simulink model "sldemo_auto_climate_elec"  (R2021b)
settings: Solver=ode23t  StartTime=0.0  StopTime=1  MaxStep=1e-4  RelTol=1e-4  AbsTol=1e-4  EnableMultiTasking=on
undefined symbols (not defined in the file or in its folder): ee
libraries: fl_lib x15, nesl_utility x10, ee_lib x9, commchan3 x3, slpidlib x1, simulink x1
(part 1 of 2)
settings Model: Creator=The MathWorks, Inc.  LastModifiedBy=dev
settings SolverCC: AutoScaleAbsTol=off  AlgebraicLoopSolver=TrustRegion
settings DataIOCC: SaveFormat=Array  ReturnWorkspaceOutputs=off  SignalLoggingName=sigsOut
settings OptimizationCC: ExpressionDepthLimit=2147483647  InitFltsAndDblsToZero=on  EfficientMapNaN2IntZero=off  LifeSpan=inf
settings DebuggingCC: AlgebraicLoopMsg=error  SaveWithParameterizedLinksMsg=none  UnderspecifiedInitializationDetection=Classic  MergeDetectMultiDrivingBlocksExec=none  SignalResolutionControl=TryResolveAllWithWarning  MultiTaskDSMMsg=warning  MultiTaskCondExecSysMsg=none  FcnCallInpInsideContextMsg=warning  StateNameClashWarn=warning  SFUnexpectedBacktrackingDiag=warning  SFNoUnconditionalDefaultTransitionDiag=warning  SFExecutionAtInitializationDiag=none  SFMachineParentedDataDiag=warning  ArithmeticOperatorsInVariantConditions=warning
settings HardwareCC: ProdBitPerPointer=32  ProdBitPerSizeT=32  ProdBitPerPtrDiffT=32  ProdLargestAtomicFloat=None  ProdIntDivRoundTo=Undefined  ProdEndianess=Unspecified  ProdWordSize=32  ProdHWDeviceType=32-bit Generic
settings ModelReferenceCC: PropagateSignalLabelsOutOfModel=off
settings SFSimCC: SimUseLocalCustomCode=off  CustomCodeUndefinedFunction=UseInterfaceOnly
settings RTWCC: RTWUseLocalCustomCode=off
settings CodeAppCC: StateflowObjectComments=on
settings GRTTargetCC: TargetFcnLib=ansi_tfl_tmw.mat  TargetLangStandard=C89/C90 (ANSI)  CombineOutputUpdateFcns=off  GRTInterface=on
settings ConfigComp: CovMetricSettings=dw  CovSaveCumulativeToWorkspaceVar=on  CovSaveSingleToWorkspaceVar=on  CovExternalEMLEnable=off
settings SimscapeCC: SimscapeLogType=all  SimscapeLogName=simlog_sldemo_auto_climate_elec  SimscapeLogLimitData=off

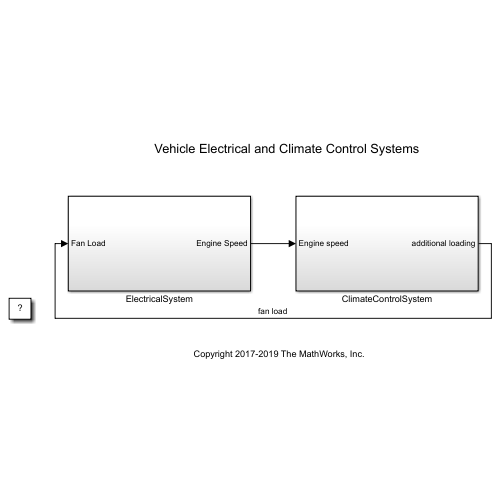
[thumbnail: Simulink's stored preview of the top-level diagram]
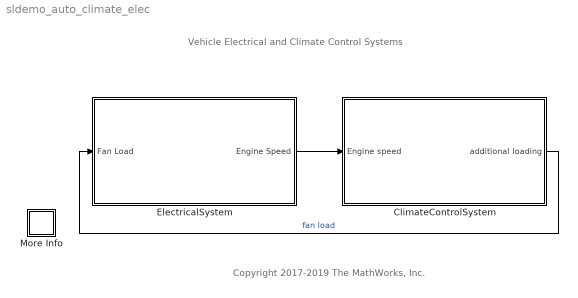
== system sldemo_auto_climate_elec ==
  note: Vehicle Electrical and Climate Control Systems
  note: Copyright 2017-2019 The MathWorks, Inc.
  ClimateControlSystem : Subsystem
  ElectricalSystem : Subsystem
  More Info : Subsystem
      settings: OpenFcn=showExample('simulink_automotive/VehicleElectricalAndClimateControlSystemsExample')
      mask Display: disp('?')
  wires:
  ElectricalSystem/1(Engine Speed) -> ClimateControlSystem/1(Engine speed)
  ClimateControlSystem/1(additional loading) -> ElectricalSystem/1(Fan Load)  "fan load"

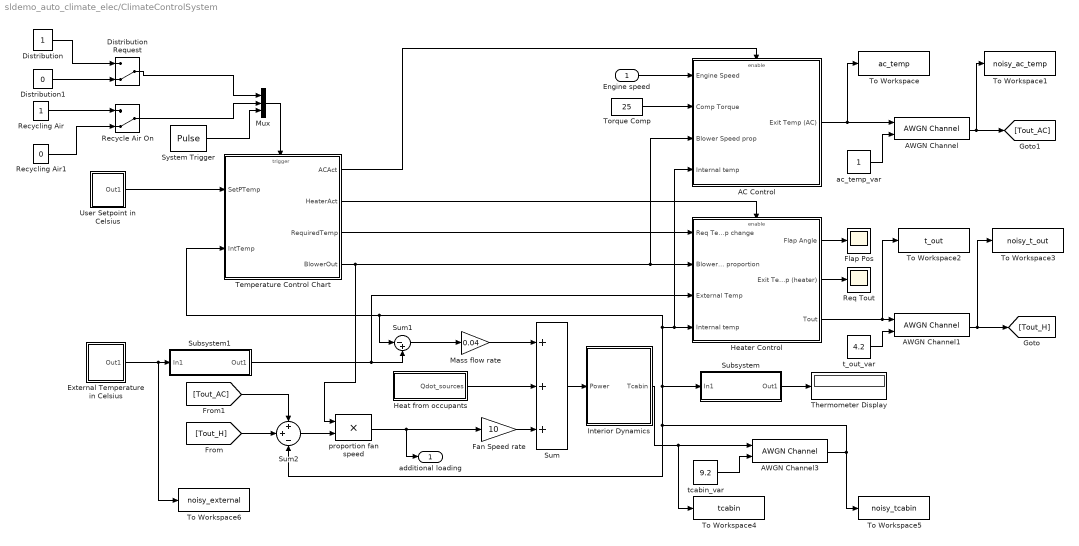
== system sldemo_auto_climate_elec/ClimateControlSystem ==
  Engine speed : Inport
  AC Control : Subsystem  TreatAsAtomicUnit=on
  AWGN Channel : commchan3/AWGN Channel  InputProcessing=Columns as channels (frame based)  seed=67  noiseMode=Variance from port  EbNodB=10  EsNodB=10  SNRdB=10  bitsPerSym=1  Ps=1  Tsym=1  variance=1
  AWGN Channel1 : commchan3/AWGN Channel  InputProcessing=Columns as channels (frame based)  seed=67  noiseMode=Variance from port  EbNodB=10  EsNodB=10  SNRdB=10  bitsPerSym=1  Ps=1  Tsym=1  variance=1
  AWGN Channel3 : commchan3/AWGN Channel  InputProcessing=Columns as channels (frame based)  seed=67  noiseMode=Variance from port  EbNodB=10  EsNodB=10  SNRdB=10  bitsPerSym=1  Ps=1  Tsym=1  variance=1
  "Distribution " : Constant
  Distribution Request : ManualSwitch  CurrentSetting=0
  "Distribution1 " : Constant  Value=0
  External Temperature in Celsius : Subsystem  mask(variable){x=18}
      mask prompts: x "Enter the external temperature"
      mask Display: disp(x);
  Fan Speed rate : Gain  Gain=10  SaturateOnIntegerOverflow=on  OutDataTypeStr=Inherit: Same as input  ParamDataTypeStr=Inherit: Same as input
  Flap Pos : Scope
  Heat from occupants : Subsystem  mask(Heat from occupants){N=1}
      mask prompts: N "Number of occupants:"
      settings: AttributesFormatString=No. of occupants: %<N>
      mask Display: disp('Heat Sources')
  Heater Control : Subsystem  TreatAsAtomicUnit=on
  Interior Dynamics : Subsystem  mask(Vehicle Cabin Dynamics){}
      mask Display: image('$imagefile') % use "Edit Image" on toolstrip to change
  Mass flow rate : Gain  Gain=0.04  SaturateOnIntegerOverflow=on  OutDataTypeStr=Inherit: Same as input  ParamDataTypeStr=Inherit: Same as input
  Mux : Mux  Inputs=3
  Recycle Air On : ManualSwitch  CurrentSetting=0
  Recycling Air : Constant
  Recycling Air1 : Constant  Value=0
  Req Tout : Scope
  Subsystem : Subsystem
      mask Display: disp('Kelvin to Celsius')
  Subsystem1 : Subsystem
      mask Display: disp('Celsius to Kelvin')
  Sum : Sum  Inputs=+++  InputSameDT=on  SaturateOnIntegerOverflow=on  OutDataTypeStr=Inherit: Same as first input
  Sum1 : Sum  Inputs=|-+  InputSameDT=on  SaturateOnIntegerOverflow=on  OutDataTypeStr=Inherit: Same as first input
  Sum2 : Sum  Inputs=++-  InputSameDT=on  SaturateOnIntegerOverflow=on  OutDataTypeStr=Inherit: Same as first input
  System Trigger : DiscretePulseGenerator  PulseType=Time based  Period=1/60  PulseWidth=50
  Temperature Control Chart : Stateflow chart  TreatAsAtomicUnit=on
  Thermometer Display : Display
  To Workspace : ToWorkspace  VariableName=ac_temp  SampleTime=-1
      settings: Save2DSignal=2-D array (concatenate along first dimension)
  To Workspace1 : ToWorkspace  VariableName=noisy_ac_temp  SampleTime=-1
      settings: Save2DSignal=2-D array (concatenate along first dimension)
  To Workspace2 : ToWorkspace  VariableName=t_out  SampleTime=-1
      settings: Save2DSignal=2-D array (concatenate along first dimension)
  To Workspace3 : ToWorkspace  VariableName=noisy_t_out  SampleTime=-1
      settings: Save2DSignal=2-D array (concatenate along first dimension)
  To Workspace4 : ToWorkspace  VariableName=tcabin  SampleTime=-1
      settings: Save2DSignal=2-D array (concatenate along first dimension)
  To Workspace5 : ToWorkspace  VariableName=noisy_tcabin  SampleTime=-1
      settings: Save2DSignal=2-D array (concatenate along first dimension)
  To Workspace6 : ToWorkspace  VariableName=noisy_external  SampleTime=-1
      settings: Save2DSignal=2-D array (concatenate along first dimension)
  Torque Comp : Constant  Value=25
  User Setpoint in Celsius : Subsystem  mask{USet=40}
      mask prompts: USet "Enter the Temperature you require"
      mask Display: disp(USet)
  ac_temp_var : Constant
  proportion fan speed : Product  InputSameDT=on  SaturateOnIntegerOverflow=on  OutDataTypeStr=Inherit: Same as first input
  t_out_var : Constant  Value=4.2
  tcabin_var : Constant  Value=9.2
  additional loading : Outport  VectorParamsAs1DForOutWhenUnconnected=off
  wires:
  Sum/1 -> Interior Dynamics/1(Power)
  Mux/1 -> Temperature Control Chart/Trigger
  Engine speed/1 -> AC Control/1(Engine Speed)
  AC Control/1(Exit Temp (AC)) -> To Workspace/1, AWGN Channel/1
  Temperature Control Chart/3(RequiredTemp) -> Heater Control/1(Req Temp change)
  Torque Comp/1 -> AC Control/2(Comp Torque)
  [Tout_AC] -> Sum2/1
  Temperature Control Chart/1(" ACAct") -> AC Control/Enable
  [Tout_H] -> Sum2/2
  Heater Control/3(Tout) -> To Workspace2/1, AWGN Channel1/1
  Heater Control/2(Exit Temp (heater)) -> Req Tout/1
  Heater Control/1(Flap Angle) -> Flap Pos/1
  Temperature Control Chart/2(" HeaterAct") -> Heater Control/Enable
  proportion fan speed/1 -> Fan Speed rate/1, additional loading/1
  Temperature Control Chart/4(BlowerOut) -> proportion fan speed/1, Heater Control/2(Blower Speed proportion), AC Control/3(Blower Speed prop)
  Sum2/1 -> proportion fan speed/2
  Fan Speed rate/1 -> Sum/3
  Subsystem1/1(Out1) -> Sum1/2, Heater Control/3(External Temp)
  Sum1/1 -> Mass flow rate/1
  Mass flow rate/1 -> Sum/1
  Heat from occupants/1(Qdot_sources) -> Sum/2
  Subsystem/1(Out1) -> Thermometer Display/1
  AWGN Channel3/1 -> To Workspace5/1, Subsystem/1(In1), Sum1/1, Temperature Control Chart/2(IntTemp), Heater Control/4(Internal temp), AC Control/4(Internal temp), Sum2/3
  System Trigger/1 -> Mux/3
  Recycle Air On/1 -> Mux/2
  Recycling Air/1 -> Recycle Air On/1
  User Setpoint in Celsius/1(Out1) -> Temperature Control Chart/1(SetPTemp)
  Recycling Air1/1 -> Recycle Air On/2
  "Distribution1 "/1 -> Distribution Request/2
  "Distribution "/1 -> Distribution Request/1
  Distribution Request/1 -> Mux/1
  AWGN Channel/1 -> To Workspace1/1, [Tout_AC]
  ac_temp_var/1 -> AWGN Channel/2
  AWGN Channel1/1 -> To Workspace3/1, [Tout_H]
  t_out_var/1 -> AWGN Channel1/2
  External Temperature in Celsius/1(Out1) -> To Workspace6/1, Subsystem1/1(In1)
  tcabin_var/1 -> AWGN Channel3/2
  Interior Dynamics/1("Tcabin ") -> AWGN Channel3/1, To Workspace4/1

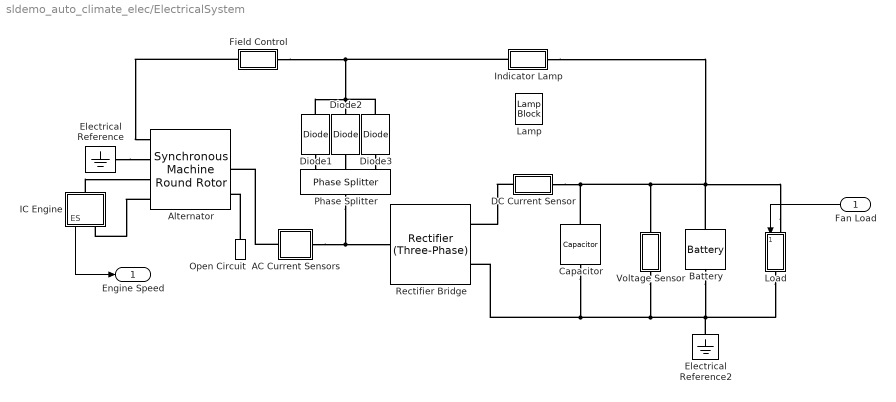
== system sldemo_auto_climate_elec/ElectricalSystem ==
  Fan Load : Inport
  AC Current Sensors : Subsystem
  Alternator : ee_lib/Electromechanical/Synchronous/Synchronous Machine Round Rotor  port_option=ee.enum.threePhasePort.composite  SRated=750 V*A  VRated=20 V  FRated=60 Hz  nPolePairs=3  param_option=ee.enum.sm.parameterization.fundamental  fieldCircuitParameterization_option=1  baseEfd=4.5 V  baseIfd=1300 A  zero_sequence=ee.enum.park.zerosequence.include  axes_param=ee.enum.rotorangle.daxis  Ladu=12.8  Laqu=12.48  L0=0.6  Ll=0.6  Ra=0.64  Lfd=1.32  Rfd=0.48  L1d=0.96  R1d=1.12  L1q=1.04  R1q=0.192  L2q=1.12  R2q=0.048  Xl=0.15  Xd=1.81  Xq=1.76  X0=0.15  Xdd=0.3  Xqd=0.65  Xddd=0.23  Xqdd=0.25  d_option=ee.enum.circuit.open  Td0d=8 s  Tdd=1.3260 s  Td0dd=0.03 s  Tddd=0.0230 s  q_option=ee.enum.circuit.open  Tq0d=1 s  Tqd=0.3693 s  Tq0dd=0.07 s  Tqdd=0.0269 s  saturation_option=0  saturation_ifd=[0, .48, .76, 1.38, 1.79]  saturation_Vag=[0, .8, 1.08, 1.31, 1.4]  initialization_option=1  source_type=ee.enum.sm.load_flow_source_type.Swing  Vmag0=1 V  Vang0=0 deg  Pt0=0 V*A  Qt0=0 V*A  minimum_pu=0.95  phase_search_range=[-30, 30] deg  gmin=1e-6 S  connection_option=int32(ee.enum.Connection.wye)  num_q_dampers=2  rotor_offset=-pi / 2 rad  pu_psid_specify=on  pu_psid_priority=High  pu_psid=0  pu_psid_nominal_specify=off  pu_psid_nominal_unit=1  pu_psid_nominal_value=1  pu_psiq_specify=on  pu_psiq_priority=High  pu_psiq=0  pu_psiq_nominal_specify=off  pu_psiq_nominal_unit=1  pu_psiq_nominal_value=1  pu_psifd_specify=on  pu_psifd_priority=High  pu_psifd=0  pu_psifd_nominal_specify=off  pu_psifd_nominal_unit=1  pu_psifd_nominal_value=1  pu_psi1d_specify=on  pu_psi1d_priority=High  pu_psi1d=0  pu_psi1d_nominal_specify=off  pu_psi1d_nominal_unit=1  pu_psi1d_nominal_value=1  pu_psi1q_specify=on  pu_psi1q_priority=High  pu_psi1q=0  pu_psi1q_nominal_specify=off  pu_psi1q_nominal_unit=1  pu_psi1q_nominal_value=1  pu_psi2q_specify=on  pu_psi2q_priority=High  pu_psi2q=0  pu_psi2q_nominal_specify=off  pu_psi2q_nominal_unit=1  pu_psi2q_nominal_value=1  angular_position_diff_specify=on  angular_position_diff_priority=High  angular_position_diff=0 deg  angular_position_diff_nominal_specify=off  angular_position_diff_nominal_unit=deg  angular_position_diff_nominal_value=1  Tmeas=298.15 K  alpha=3.93e-3 1/K  stator_thermal_mass=100 J/K  rotor_thermal_mass=200 J/K  temperatureA_specify=off  temperatureA_priority=High  temperatureA=25 degC  temperatureA_nominal_specify=off  temperatureA_nominal_unit=degC  temperatureA_nominal_value=1  temperatureB_specify=off  temperatureB_priority=High  temperatureB=25 degC  temperatureB_nominal_specify=off  temperatureB_nominal_unit=degC  temperatureB_nominal_value=1  temperatureC_specify=off  temperatureC_priority=High  temperatureC=25 degC  temperatureC_nominal_specify=off  temperatureC_nominal_unit=degC  temperatureC_nominal_value=1  temperatureR_specify=off  temperatureR_priority=High  temperatureR=25 degC  temperatureR_nominal_specify=off  temperatureR_nominal_unit=degC  temperatureR_nominal_value=1
      settings: SourceProductBaseCode=PS  InternalSimscapePortConfiguration="{\"Bottom\":[],\"Left\":[{\"id\":\"fd_p\",\"label\":\"fd+\",\"type\":\"foundation.electrical.electrical\"},{\"id\":\"fd_n\",\"label\":\"fd-\",\"type\":\"foundation.electrical.electrical\"},{\"id\":\"R\",\"label\":\"R\",\"type\":\"foundation.mechanical.rotational.rotational\"},{\"id\":\"C\",\"label\":\"C\",\"type\":\"foundation.mechanical.rotational.rotational\"}],\"Right\":[{\"id\":\"pu_output\",\"label\":\"pu\",\"type\":\"output\"},{\"id\":\"N\",\"label\":\"~\",\"type\":\"foundation.electrical.three_phase\"},{\"id\":\"n\",\"label\":\"n\",\"type\":\"foundation.electrical.electrical\"}],\"Top\":[]}"
  Battery : ee_lib/Sources/Battery  Vnom=12 V  prm_dir=1  R1_dis=2 Ohm  R1_ch=2 Ohm  R1=0.5 Ohm  prm_AH=2  AH=50 hr*A  V1=11.5 V  AH1=25 hr*A  prm_R2=1  R2=2000 Ohm  prm_dyn=1  Rp1=0.005 Ohm  tau1=30 s  Rp2=0.005 Ohm  tau2=30 s  Rp3=0.005 Ohm  tau3=30 s  Rp4=0.005 Ohm  tau4=30 s  Rp5=0.005 Ohm  tau5=30 s  prm_fade=1  N_fade=100  AH_fade=45 hr*A  R1_fade=2.02 Ohm  R1_ch_fade=2.02 Ohm  V1_fade=10.35 V  prm_age=1  prm_age_OCV=1  OCV_age=0.9  SOC_age=60  delta_time_age_vec=[0] d  temperature_age_vec=[273] K  OCV_scaling_age=2.2134e6  OCV_offset_age=1.632e6  temp_exp_age=0.515833569 V  t_exp_age=0.75  i_specify=off  i_priority=None  i=0 A  i_nominal_specify=off  i_nominal_unit=A  i_nominal_value=1  v_specify=off  v_priority=None  v=0 V  v_nominal_specify=off  v_nominal_unit=V  v_nominal_value=1  charge_specify=on  charge_priority=High  charge=50*0.80 hr*A  charge_nominal_specify=off  charge_nominal_unit=hr*A  charge_nominal_value=1  num_cycles_specify=off  num_cycles_priority=High  num_cycles=0  num_cycles_nominal_specify=off  num_cycles_nominal_unit=1  num_cycles_nominal_value=1  Tmeas=298.15 K  Tmeas_age=298.15 K  Vnom_T2=12 V  R1_T2=2.2 Ohm  R1_T2_dis=2.2 Ohm  R1_T2_ch=2.2 Ohm  V1_T2=11.4 V  R2_T2=2200 Ohm  Rp1_T2=0.005 Ohm  tau1_T2=30 s  Rp2_T2=0.005 Ohm  tau2_T2=30 s  Rp3_T2=0.005 Ohm  tau3_T2=30 s  Rp4_T2=0.005 Ohm  tau4_T2=30 s  Rp5_T2=0.005 Ohm  tau5_T2=30 s  Tmeas2=273.15 K  thermal_mass=30000 J/K  temperature_specify=off  temperature_priority=High  temperature=298.15 K  temperature_nominal_specify=off  temperature_nominal_unit=K  temperature_nominal_value=1
  Capacitor : fl_lib/Electrical/Electrical Elements/Capacitor  c=50e-6 F  r=0 Ohm  g=1e-6 1/Ohm  i_specify=off  i_priority=None  i=0 A  i_nominal_specify=off  i_nominal_unit=A  i_nominal_value=1  v_specify=off  v_priority=None  v=0 V  v_nominal_specify=off  v_nominal_unit=V  v_nominal_value=1  vc_specify=on  vc_priority=High  vc=12 V  vc_nominal_specify=off  vc_nominal_unit=V  vc_nominal_value=1
  DC Current Sensor : Subsystem
  Diode1 : ee_lib/Semiconductors & Converters/Diode  ModelType=ee.enum.diode.modelType.pwl  TableType=ee.enum.diode.tableType.IfMat  IfMat=[.07, .12, .19, 1.75, 4.24, 7.32, 11.2; .16, .3, .72, 2.14, 5.02, 8.35, 13.12] A  VfMat=[.9, 1.15, 1.25, 1.5, 1.75, 2.17, 2.6, 2.85; .58, .68, .75, 1.1, 1.38, 1.77, 2.27, 2.7] V  TjVec=[25, 125] degC  VfVec=[.5, .7, .9, 1.3, 1.7, 2.1, 2.5] V  IfVec=[.1, .2, .5, 1, 2, 4, 7, 10] A  Vf=0.8 V  Ron=0.001 Ohm  Goff=1e-5 1/Ohm  prmExp=ee.enum.diode.expParam.useTwo  I12=[.0137, .545] A  V12=[.6, .7] V  RS=0 Ohm  Tmeas=25 degC  IS=1e-12 A  ec=1  I1=0.0137 A  V1=0.6 V  N_series=1  N_parallel=1  Rz=0.3 Ohm  BV=inf V  C_param=ee.enum.diode.capParam.fixed  CJ=0 pF  CJ0=5 pF  Vvec=[.1, 10, 100] V  Cvec=[3.5, 1, .4] pF  VJ=1 V  Mgrad=0.5  FC=0.5  Q_param=ee.enum.diode.recoveryParam.off  iRM=-7.15 A  iF=4 A  didt=-750 A/us  trr_factor=3  trr=115 ns  Qrr=1500 s*uA  Vr=-600 V  Ls=150 nH  Erec=0.03 J  TT=50 ns  tau=100 ns  T_param=ee.enum.diode.temperatureParam.off  Tdevice=25 degC  I1_T2=0.245 A  V1_T2=0.5 V  IS_T2=1.25e-7 A  Tmeas2=125 degC  XTI_param=ee.enum.diode.xtiParam.pn  XTI=3  EG_param=ee.enum.diode.egapParam.material_si  EG=1.11 eV  dBVdT=0 V/K  enable_faults=simscape.enum.onoff.off  fault_action=simscape.enum.assert.action.none  fault_types=ee.enum.diode.faults.open  tau_fault=1e-3 s  IfMat_faulted=[.07, .12, .19, 1.75, 4.24, 7.32, 11.2; .16, .3, .72, 2.14, 4.02, 6.35, 9.12] A  VfMat_faulted=[.9, 1.15, 1.25, 1.5, 1.75, 2.17, 2.6, 2.85; .58, .68, .75, 1.1, 1.38, 1.77, 2.27, 2.7] V  VfVec_faulted=[.5, .7, .9, 1.3, 1.7, 2.1, 2.5] V  IfVec_faulted=[.1, .2, .5, 1, 2, 4, 7, 10] A  Ropen_faulted=1000 Ohm  Gshort_faulted=1000 1/Ohm  Vf_faulted=0.6 V  Ron_faulted=0.3 Ohm  Goff_faulted=1e-8 S  I12_faulted=[.0137, .545] A  V12_faulted=[.6, .7] V  IS_faulted=1e-12 A  ec_faulted=1  I1_faulted=0.0137 A  V1_faulted=0.6 V  RS_faulted=0 Ohm  Rz_faulted=0.3 Ohm  BV_faulted=inf V  Cscale_faulted=100  enable_temporal_fault=simscape.enum.onoff.off  t_fault=inf s  enable_behavioral_fault=simscape.enum.onoff.off  max_permissible_voltage=inf V  n_fail_on_voltage=1  max_permissible_current=inf A  t_fail_on_current=1 s  max_permissible_dVdt=inf V/s  i_specify=off  i_priority=None  i=0 A  i_nominal_specify=off  i_nominal_unit=A  i_nominal_value=1  v_specify=off  v_priority=None  v=0 V  v_nominal_specify=off  v_nominal_unit=V  v_nominal_value=1  i_diode_specify=off  i_diode_priority=None  i_diode=0 A  i_diode_nominal_specify=off  i_diode_nominal_unit=A  i_diode_nominal_value=1  v_diode_specify=off  v_diode_priority=None  v_diode=0 V  v_diode_nominal_specify=off  v_diode_nominal_unit=V  v_diode_nominal_value=1  i_capacitor_specify=off  i_capacitor_priority=None  i_capacitor=0 A  i_capacitor_nominal_specify=off  i_capacitor_nominal_unit=A  i_capacitor_nominal_value=1  v_capacitor_specify=off  v_capacitor_priority=None  v_capacitor=0 V  v_capacitor_nominal_specify=off  v_capacitor_nominal_unit=V  v_capacitor_nominal_value=1  power_dissipated_specify=off  power_dissipated_priority=None  power_dissipated=0 W  power_dissipated_nominal_specify=off  power_dissipated_nominal_unit=W  power_dissipated_nominal_value=1  max_permissible_temperature=inf K  t_fail_on_temperature=1 s  thermal_network_parameterization=ee.enum.thermalNetworkTopology.junctionCase  Rth=[0, 10] K/W  Rth_Cauer=[1, 3, 10] K/W  Rth_Foster=[4, 6] K/W  thermal_mass_parameterization=ee.enum.thermalNetwork.timeconstant  thermal_mass=[0, 1] J/K  thermal_mass_Cauer=[.1, .3, 1] J/K  thermal_mass_Foster=[1.5, 3] J/K  thermal_time_constant=[0, 10] s  thermal_time_constant_Cauer=[1, 3, 10] s  thermal_time_constant_Foster=[6, 18] s  thermal_mass_initial_temperatures=[25, 25] degC  thermal_mass_initial_temperatures_Cauer=[25, 25, 25] degC  steadyState_Foster=simscape.enum.onoff.on  Tvec_initial_Foster=[25, 25, 25, 25] degC
  Diode2 : ee_lib/Semiconductors & Converters/Diode  ModelType=ee.enum.diode.modelType.pwl  TableType=ee.enum.diode.tableType.IfMat  IfMat=[.07, .12, .19, 1.75, 4.24, 7.32, 11.2; .16, .3, .72, 2.14, 5.02, 8.35, 13.12] A  VfMat=[.9, 1.15, 1.25, 1.5, 1.75, 2.17, 2.6, 2.85; .58, .68, .75, 1.1, 1.38, 1.77, 2.27, 2.7] V  TjVec=[25, 125] degC  VfVec=[.5, .7, .9, 1.3, 1.7, 2.1, 2.5] V  IfVec=[.1, .2, .5, 1, 2, 4, 7, 10] A  Vf=0.8 V  Ron=0.001 Ohm  Goff=1e-5 1/Ohm  prmExp=ee.enum.diode.expParam.useTwo  I12=[.0137, .545] A  V12=[.6, .7] V  RS=0 Ohm  Tmeas=25 degC  IS=1e-12 A  ec=1  I1=0.0137 A  V1=0.6 V  N_series=1  N_parallel=1  Rz=0.3 Ohm  BV=inf V  C_param=ee.enum.diode.capParam.fixed  CJ=0 pF  CJ0=5 pF  Vvec=[.1, 10, 100] V  Cvec=[3.5, 1, .4] pF  VJ=1 V  Mgrad=0.5  FC=0.5  Q_param=ee.enum.diode.recoveryParam.off  iRM=-7.15 A  iF=4 A  didt=-750 A/us  trr_factor=3  trr=115 ns  Qrr=1500 s*uA  Vr=-600 V  Ls=150 nH  Erec=0.03 J  TT=50 ns  tau=100 ns  T_param=ee.enum.diode.temperatureParam.off  Tdevice=25 degC  I1_T2=0.245 A  V1_T2=0.5 V  IS_T2=1.25e-7 A  Tmeas2=125 degC  XTI_param=ee.enum.diode.xtiParam.pn  XTI=3  EG_param=ee.enum.diode.egapParam.material_si  EG=1.11 eV  dBVdT=0 V/K  enable_faults=simscape.enum.onoff.off  fault_action=simscape.enum.assert.action.none  fault_types=ee.enum.diode.faults.open  tau_fault=1e-3 s  IfMat_faulted=[.07, .12, .19, 1.75, 4.24, 7.32, 11.2; .16, .3, .72, 2.14, 4.02, 6.35, 9.12] A  VfMat_faulted=[.9, 1.15, 1.25, 1.5, 1.75, 2.17, 2.6, 2.85; .58, .68, .75, 1.1, 1.38, 1.77, 2.27, 2.7] V  VfVec_faulted=[.5, .7, .9, 1.3, 1.7, 2.1, 2.5] V  IfVec_faulted=[.1, .2, .5, 1, 2, 4, 7, 10] A  Ropen_faulted=1000 Ohm  Gshort_faulted=1000 1/Ohm  Vf_faulted=0.6 V  Ron_faulted=0.3 Ohm  Goff_faulted=1e-8 S  I12_faulted=[.0137, .545] A  V12_faulted=[.6, .7] V  IS_faulted=1e-12 A  ec_faulted=1  I1_faulted=0.0137 A  V1_faulted=0.6 V  RS_faulted=0 Ohm  Rz_faulted=0.3 Ohm  BV_faulted=inf V  Cscale_faulted=100  enable_temporal_fault=simscape.enum.onoff.off  t_fault=inf s  enable_behavioral_fault=simscape.enum.onoff.off  max_permissible_voltage=inf V  n_fail_on_voltage=1  max_permissible_current=inf A  t_fail_on_current=1 s  max_permissible_dVdt=inf V/s  i_specify=off  i_priority=None  i=0 A  i_nominal_specify=off  i_nominal_unit=A  i_nominal_value=1  v_specify=off  v_priority=None  v=0 V  v_nominal_specify=off  v_nominal_unit=V  v_nominal_value=1  i_diode_specify=off  i_diode_priority=None  i_diode=0 A  i_diode_nominal_specify=off  i_diode_nominal_unit=A  i_diode_nominal_value=1  v_diode_specify=off  v_diode_priority=None  v_diode=0 V  v_diode_nominal_specify=off  v_diode_nominal_unit=V  v_diode_nominal_value=1  i_capacitor_specify=off  i_capacitor_priority=None  i_capacitor=0 A  i_capacitor_nominal_specify=off  i_capacitor_nominal_unit=A  i_capacitor_nominal_value=1  v_capacitor_specify=off  v_capacitor_priority=None  v_capacitor=0 V  v_capacitor_nominal_specify=off  v_capacitor_nominal_unit=V  v_capacitor_nominal_value=1  power_dissipated_specify=off  power_dissipated_priority=None  power_dissipated=0 W  power_dissipated_nominal_specify=off  power_dissipated_nominal_unit=W  power_dissipated_nominal_value=1  max_permissible_temperature=inf K  t_fail_on_temperature=1 s  thermal_network_parameterization=ee.enum.thermalNetworkTopology.junctionCase  Rth=[0, 10] K/W  Rth_Cauer=[1, 3, 10] K/W  Rth_Foster=[4, 6] K/W  thermal_mass_parameterization=ee.enum.thermalNetwork.timeconstant  thermal_mass=[0, 1] J/K  thermal_mass_Cauer=[.1, .3, 1] J/K  thermal_mass_Foster=[1.5, 3] J/K  thermal_time_constant=[0, 10] s  thermal_time_constant_Cauer=[1, 3, 10] s  thermal_time_constant_Foster=[6, 18] s  thermal_mass_initial_temperatures=[25, 25] degC  thermal_mass_initial_temperatures_Cauer=[25, 25, 25] degC  steadyState_Foster=simscape.enum.onoff.on  Tvec_initial_Foster=[25, 25, 25, 25] degC
  Diode3 : ee_lib/Semiconductors & Converters/Diode  ModelType=ee.enum.diode.modelType.pwl  TableType=ee.enum.diode.tableType.IfMat  IfMat=[.07, .12, .19, 1.75, 4.24, 7.32, 11.2; .16, .3, .72, 2.14, 5.02, 8.35, 13.12] A  VfMat=[.9, 1.15, 1.25, 1.5, 1.75, 2.17, 2.6, 2.85; .58, .68, .75, 1.1, 1.38, 1.77, 2.27, 2.7] V  TjVec=[25, 125] degC  VfVec=[.5, .7, .9, 1.3, 1.7, 2.1, 2.5] V  IfVec=[.1, .2, .5, 1, 2, 4, 7, 10] A  Vf=0.8 V  Ron=0.001 Ohm  Goff=1e-5 1/Ohm  prmExp=ee.enum.diode.expParam.useTwo  I12=[.0137, .545] A  V12=[.6, .7] V  RS=0 Ohm  Tmeas=25 degC  IS=1e-12 A  ec=1  I1=0.0137 A  V1=0.6 V  N_series=1  N_parallel=1  Rz=0.3 Ohm  BV=inf V  C_param=ee.enum.diode.capParam.fixed  CJ=0 pF  CJ0=5 pF  Vvec=[.1, 10, 100] V  Cvec=[3.5, 1, .4] pF  VJ=1 V  Mgrad=0.5  FC=0.5  Q_param=ee.enum.diode.recoveryParam.off  iRM=-7.15 A  iF=4 A  didt=-750 A/us  trr_factor=3  trr=115 ns  Qrr=1500 s*uA  Vr=-600 V  Ls=150 nH  Erec=0.03 J  TT=50 ns  tau=100 ns  T_param=ee.enum.diode.temperatureParam.off  Tdevice=25 degC  I1_T2=0.245 A  V1_T2=0.5 V  IS_T2=1.25e-7 A  Tmeas2=125 degC  XTI_param=ee.enum.diode.xtiParam.pn  XTI=3  EG_param=ee.enum.diode.egapParam.material_si  EG=1.11 eV  dBVdT=0 V/K  enable_faults=simscape.enum.onoff.off  fault_action=simscape.enum.assert.action.none  fault_types=ee.enum.diode.faults.open  tau_fault=1e-3 s  IfMat_faulted=[.07, .12, .19, 1.75, 4.24, 7.32, 11.2; .16, .3, .72, 2.14, 4.02, 6.35, 9.12] A  VfMat_faulted=[.9, 1.15, 1.25, 1.5, 1.75, 2.17, 2.6, 2.85; .58, .68, .75, 1.1, 1.38, 1.77, 2.27, 2.7] V  VfVec_faulted=[.5, .7, .9, 1.3, 1.7, 2.1, 2.5] V  IfVec_faulted=[.1, .2, .5, 1, 2, 4, 7, 10] A  Ropen_faulted=1000 Ohm  Gshort_faulted=1000 1/Ohm  Vf_faulted=0.6 V  Ron_faulted=0.3 Ohm  Goff_faulted=1e-8 S  I12_faulted=[.0137, .545] A  V12_faulted=[.6, .7] V  IS_faulted=1e-12 A  ec_faulted=1  I1_faulted=0.0137 A  V1_faulted=0.6 V  RS_faulted=0 Ohm  Rz_faulted=0.3 Ohm  BV_faulted=inf V  Cscale_faulted=100  enable_temporal_fault=simscape.enum.onoff.off  t_fault=inf s  enable_behavioral_fault=simscape.enum.onoff.off  max_permissible_voltage=inf V  n_fail_on_voltage=1  max_permissible_current=inf A  t_fail_on_current=1 s  max_permissible_dVdt=inf V/s  i_specify=off  i_priority=None  i=0 A  i_nominal_specify=off  i_nominal_unit=A  i_nominal_value=1  v_specify=off  v_priority=None  v=0 V  v_nominal_specify=off  v_nominal_unit=V  v_nominal_value=1  i_diode_specify=off  i_diode_priority=None  i_diode=0 A  i_diode_nominal_specify=off  i_diode_nominal_unit=A  i_diode_nominal_value=1  v_diode_specify=off  v_diode_priority=None  v_diode=0 V  v_diode_nominal_specify=off  v_diode_nominal_unit=V  v_diode_nominal_value=1  i_capacitor_specify=off  i_capacitor_priority=None  i_capacitor=0 A  i_capacitor_nominal_specify=off  i_capacitor_nominal_unit=A  i_capacitor_nominal_value=1  v_capacitor_specify=off  v_capacitor_priority=None  v_capacitor=0 V  v_capacitor_nominal_specify=off  v_capacitor_nominal_unit=V  v_capacitor_nominal_value=1  power_dissipated_specify=off  power_dissipated_priority=None  power_dissipated=0 W  power_dissipated_nominal_specify=off  power_dissipated_nominal_unit=W  power_dissipated_nominal_value=1  max_permissible_temperature=inf K  t_fail_on_temperature=1 s  thermal_network_parameterization=ee.enum.thermalNetworkTopology.junctionCase  Rth=[0, 10] K/W  Rth_Cauer=[1, 3, 10] K/W  Rth_Foster=[4, 6] K/W  thermal_mass_parameterization=ee.enum.thermalNetwork.timeconstant  thermal_mass=[0, 1] J/K  thermal_mass_Cauer=[.1, .3, 1] J/K  thermal_mass_Foster=[1.5, 3] J/K  thermal_time_constant=[0, 10] s  thermal_time_constant_Cauer=[1, 3, 10] s  thermal_time_constant_Foster=[6, 18] s  thermal_mass_initial_temperatures=[25, 25] degC  thermal_mass_initial_temperatures_Cauer=[25, 25, 25] degC  steadyState_Foster=simscape.enum.onoff.on  Tvec_initial_Foster=[25, 25, 25, 25] degC
  Electrical Reference : fl_lib/Electrical/Electrical Elements/Electrical Reference
  Electrical Reference2 : fl_lib/Electrical/Electrical Elements/Electrical Reference
  Field Control : Subsystem
  IC Engine : Subsystem
  Indicator Lamp : Subsystem
  Lamp : LampBlock  LabelPosition=Hide
  Load : Subsystem
  Open Circuit : fl_lib/Electrical/Electrical Elements/Open Circuit  v_specify=off  v_priority=None  v=0 V  v_nominal_specify=off  v_nominal_unit=V  v_nominal_value=1
      settings: SourceProductBaseCode=SS
  Phase Splitter : ee_lib/Connectors & References/Phase Splitter
      settings: SourceProductBaseCode=PS
  Rectifier Bridge : ee_lib/Semiconductors & Converters/Converters/Rectifier (Three-Phase)  port_option=ee.enum.threePhasePort.composite  Vf=0.8 V  Ron=0.001 Ohm  Goff=1e-5 1/Ohm  model_dynamics=ee.enum.converters.diode.nodynamics  C=50 nF  iRM=-235 A  iF=300 A  idot=-50 A/us  trr_param=1  trr_factor=3  trr=15 us  Qrr=1500 s*uA
      settings: SourceProductBaseCode=PS  InternalSimscapePortConfiguration="{\"Bottom\":[],\"Left\":[{\"id\":\"N\",\"label\":\"~\",\"type\":\"foundation.electrical.three_phase\"}],\"Right\":[{\"id\":\"p\",\"label\":\"+\",\"type\":\"foundation.electrical.electrical\"},{\"id\":\"n\",\"label\":\"-\",\"type\":\"foundation.electrical.electrical\"}],\"Top\":[]}"
  Voltage Sensor : Subsystem
  Engine Speed : Outport  InitialOutput=0  VectorParamsAs1DForOutWhenUnconnected=off
  wires:
  IC Engine/1(ES) -> Engine Speed/1
  Fan Load/1 -> Load/1(FL)
  connections:
  Capacitor/RConn1 -- Electrical Reference2/LConn1 -- Load/RConn1 -- Battery/RConn1 -- Voltage Sensor/RConn1 -- Rectifier Bridge/RConn2
  Diode2/RConn1 -- Diode3/RConn1 -- Indicator Lamp/LConn1 -- Field Control/LConn1 -- Diode1/RConn1
  Phase Splitter/LConn1 -- AC Current Sensors/RConn1 -- Rectifier Bridge/LConn1
  Load/LConn1 -- Capacitor/LConn1 -- DC Current Sensor/RConn1 -- Voltage Sensor/LConn1 -- Indicator Lamp/RConn1 -- Battery/LConn1
  Open Circuit/LConn1 -- Alternator/RConn3
  Diode3/LConn1 -- Phase Splitter/RConn3
  DC Current Sensor/LConn1 -- Rectifier Bridge/RConn1
  IC Engine/LConn1 -- Alternator/LConn3
  AC Current Sensors/LConn1 -- Alternator/RConn2
  Alternator/LConn4 -- IC Engine/RConn1
  Electrical Reference/LConn1 -- Alternator/LConn2
  Field Control/RConn1 -- Alternator/LConn1
  Diode2/LConn1 -- Phase Splitter/RConn2
  Diode1/LConn1 -- Phase Splitter/RConn1

== system sldemo_auto_climate_elec/More Info ==

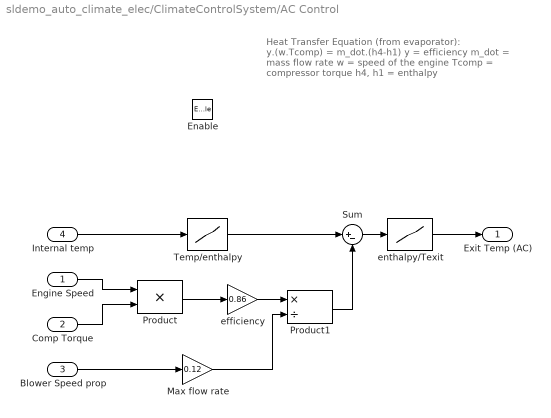
== system sldemo_auto_climate_elec/ClimateControlSystem/AC Control ==
  note: Heat Transfer Equation (from evaporator):
      |
      | y.(w.Tcomp) = m_dot.(h4-h1)
      |
      | y = efficiency
      | m_dot = mass flow rate
      | w = speed of the engine
      | Tcomp = compressor torque
      | h4, h1 = enthalpy
  Engine Speed : Inport
  Comp Torque : Inport  Port=2
  Blower Speed prop : Inport  Port=3
  Internal temp : Inport  Port=4
  Enable : EnablePort  StatesWhenEnabling=reset  PropagateVarSize=During execution  ZeroCross=off
  Max flow rate : Gain  Gain=0.12  SaturateOnIntegerOverflow=on  OutDataTypeStr=Inherit: Same as input  ParamDataTypeStr=Inherit: Same as input
  Product : Product  InputSameDT=on  SaturateOnIntegerOverflow=on  OutDataTypeStr=Inherit: Same as first input
  Product1 : Product  Inputs=*/  InputSameDT=on  SaturateOnIntegerOverflow=on  OutDataTypeStr=Inherit: Same as first input
  Sum : Sum  Inputs=|+-  InputSameDT=on  SaturateOnIntegerOverflow=on  OutDataTypeStr=Inherit: Same as first input
  Temp/enthalpy : Lookup_n-D  NumberOfTableDimensions=1  BreakpointsForDimension1=[220 230 240 250 260 270 280 285 290 295 300 305 310 315 320]  Table=[219.97 230.02 240.02 250.05 260.09 270.11 280.13 285.14 290.16 295.17 300.19 305.22 310.24 315.27 320.29]  SaturateOnIntegerOverflow=on  InputSameDT=on
  efficiency : Gain  Gain=0.86  SaturateOnIntegerOverflow=on  OutDataTypeStr=Inherit: Same as input  ParamDataTypeStr=Inherit: Same as input
  enthalpy/Texit : Lookup_n-D  NumberOfTableDimensions=1  BreakpointsForDimension1=[219.97 230.02 240.02 250.05 260.09 270.11 280.13 285.14 290.16 295.17 300.19 305.22 310.24 315.27 320.29]  Table=[220 230 240 250 260 270 280 285 290 295 300 305 310 315 320]  SaturateOnIntegerOverflow=on  InputSameDT=on
  Exit Temp (AC) : Outport  OutputWhenDisabled=reset  InitialOutput=0  VectorParamsAs1DForOutWhenUnconnected=off
  wires:
  Engine Speed/1 -> Product/1
  Comp Torque/1 -> Product/2
  Product/1 -> efficiency/1
  efficiency/1 -> Product1/1
  Blower Speed prop/1 -> Max flow rate/1
  Max flow rate/1 -> Product1/2
  enthalpy/Texit/1 -> Exit Temp (AC)/1
  Internal temp/1 -> Temp/enthalpy/1
  Temp/enthalpy/1 -> Sum/1
  Product1/1 -> Sum/2
  Sum/1 -> enthalpy/Texit/1

== system sldemo_auto_climate_elec/ClimateControlSystem/External Temperature in Celsius ==
  External Temp : Constant  Value=x
  Temp Limits : Saturate  UpperLimit=100  LowerLimit=-99
  Out1 : Outport  VectorParamsAs1DForOutWhenUnconnected=off
  wires:
  External Temp/1 -> Temp Limits/1
  Temp Limits/1 -> Out1/1

== system sldemo_auto_climate_elec/ClimateControlSystem/Heat from occupants ==
  No of occupants : Gain  Gain=N  SaturateOnIntegerOverflow=on  OutDataTypeStr=Inherit: Same as input  ParamDataTypeStr=Inherit: Same as input
  Power per occupant [W] : Constant  Value=100
  Qdot_sources : Outport  VectorParamsAs1DForOutWhenUnconnected=off
  wires:
  No of occupants/1 -> Qdot_sources/1  "Qdot_sources"
  Power per occupant [W]/1 -> No of occupants/1

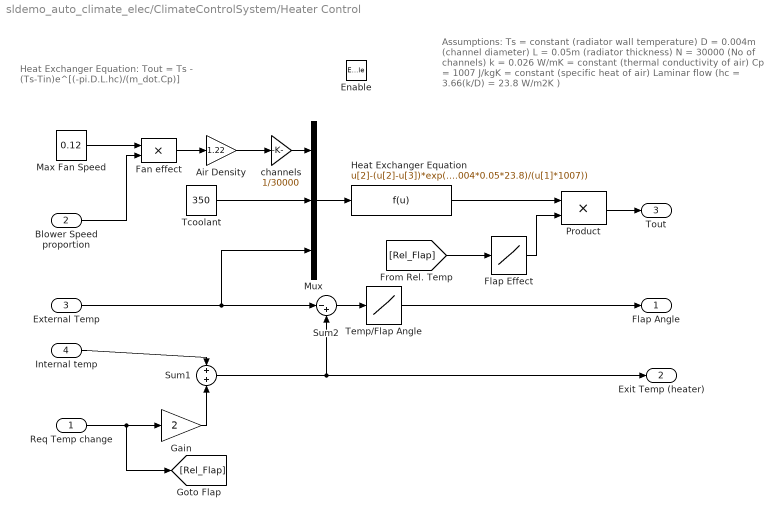
== system sldemo_auto_climate_elec/ClimateControlSystem/Heater Control ==
  note: Heat Exchanger Equation:
      | Tout = Ts - (Ts-Tin)e^[(-pi.D.L.hc)/(m_dot.Cp)]
  note: Assumptions:
      | Ts = constant (radiator wall temperature)
      | D = 0.004m (channel diameter)
      | L = 0.05m (radiator thickness)
      | N = 30000 (No of channels)
      |
      | k = 0.026 W/mK = constant (thermal conductivity of air)
      | Cp = 1007 J/kgK = constant (specific heat of air)
      | Laminar flow (hc = 3.66(k/D) = 23.8 W/m2K )
  Req Temp change : Inport
  Blower Speed proportion : Inport  Port=2
  External Temp : Inport  Port=3
  Internal temp : Inport  Port=4
  Enable : EnablePort  StatesWhenEnabling=reset  PropagateVarSize=During execution  ZeroCross=off
  Air Density : Gain  Gain=1.22  SaturateOnIntegerOverflow=on  OutDataTypeStr=Inherit: Same as input  ParamDataTypeStr=Inherit: Same as input
  Fan effect : Product  InputSameDT=on  SaturateOnIntegerOverflow=on  OutDataTypeStr=Inherit: Same as first input
  Flap Effect : Lookup_n-D  NumberOfTableDimensions=1  BreakpointsForDimension1="[0 3 5 10 50  90 100 200 ]"  Table="[0 300 100  10 10  10 3 1]"  SaturateOnIntegerOverflow=on  InputSameDT=on
  Gain : Gain  Gain=2  SaturateOnIntegerOverflow=on  OutDataTypeStr=Inherit: Same as input  ParamDataTypeStr=Inherit: Same as input
  Heat Exchanger Equation : Fcn  Expr=u[2]-(u[2]-u[3])*exp(-(pi*0.004*0.05*23.8)/(u[1]*1007))
  Max Fan Speed : Constant  Value=0.12
  Mux : Mux  Inputs=3
  Product : Product  InputSameDT=on  SaturateOnIntegerOverflow=on  OutDataTypeStr=Inherit: Same as first input
  Sum1 : Sum  InputSameDT=on  SaturateOnIntegerOverflow=on  OutDataTypeStr=Inherit: Same as first input
  Sum2 : Sum  Inputs=|-+  InputSameDT=on  SaturateOnIntegerOverflow=on  OutDataTypeStr=Inherit: Same as first input
  "Tcoolant " : Constant  Value=350
  Temp/Flap Angle : Lookup_n-D  NumberOfTableDimensions=1  BreakpointsForDimension1=[0 10 20 30 40 50 60 75 100 200]  Table=[0 20 30 45 60 75 90 90 90 90]  SaturateOnIntegerOverflow=on  InputSameDT=on
  channels : Gain  Gain=1/30000  SaturateOnIntegerOverflow=on  OutDataTypeStr=Inherit: Same as input  ParamDataTypeStr=Inherit: Same as input
  Flap Angle : Outport  OutputWhenDisabled=reset  InitialOutput=0  VectorParamsAs1DForOutWhenUnconnected=off
  Exit Temp (heater) : Outport  Port=2  OutputWhenDisabled=reset  InitialOutput=0  VectorParamsAs1DForOutWhenUnconnected=off
  Tout : Outport  Port=3  OutputWhenDisabled=reset  InitialOutput=0  VectorParamsAs1DForOutWhenUnconnected=off
  wires:
  [Rel_Flap] -> Flap Effect/1
  Flap Effect/1 -> Product/2
  Req Temp change/1 -> [Rel_Flap], Gain/1
  Sum1/1 -> Sum2/2, Exit Temp (heater)/1
  Gain/1 -> Sum1/2
  Internal temp/1 -> Sum1/1
  Sum2/1 -> Temp/Flap Angle/1
  Temp/Flap Angle/1 -> Flap Angle/1
  Product/1 -> Tout/1
  "Tcoolant "/1 -> Mux/2
  channels/1 -> Mux/1
  Air Density/1 -> channels/1
  Mux/1 -> Heat Exchanger Equation/1
  Fan effect/1 -> Air Density/1
  Max Fan Speed/1 -> Fan effect/1
  Blower Speed proportion/1 -> Fan effect/2
  External Temp/1 -> Sum2/1, Mux/3
  Heat Exchanger Equation/1 -> Product/1

== system sldemo_auto_climate_elec/ClimateControlSystem/Interior Dynamics ==
  Power : Inport
  Tcabin : Integrator  InitialCondition=291  ZeroCross=off
  dT/dt = Pnet/(pVCp) p = 1.22 kg/m3 V = 2.5 m3 Cp = 1007 J/kgK : Gain  Gain=(1/3071)  SaturateOnIntegerOverflow=on  OutDataTypeStr=Inherit: Same as input  ParamDataTypeStr=Inherit: Same as input
  "Tcabin " : Outport  VectorParamsAs1DForOutWhenUnconnected=off
  wires:
  Tcabin/1 -> "Tcabin "/1  "Tcabin [K]"
  Power/1 -> dT/dt = Pnet/(pVCp) p = 1.22 kg/m3 V = 2.5 m3 Cp = 1007 J/kgK/1
  dT/dt = Pnet/(pVCp) p = 1.22 kg/m3 V = 2.5 m3 Cp = 1007 J/kgK/1 -> Tcabin/1

== system sldemo_auto_climate_elec/ClimateControlSystem/Subsystem ==
  In1 : Inport
  Constant : Constant  Value=273
  Sum1 : Sum  Inputs=|-+  InputSameDT=on  SaturateOnIntegerOverflow=on  OutDataTypeStr=Inherit: Same as first input
  Out1 : Outport  VectorParamsAs1DForOutWhenUnconnected=off
  wires:
  Constant/1 -> Sum1/1
  In1/1 -> Sum1/2
  Sum1/1 -> Out1/1

== system sldemo_auto_climate_elec/ClimateControlSystem/Subsystem1 ==
  In1 : Inport
  Constant : Constant  Value=273
  Sum1 : Sum  Inputs=|++  InputSameDT=on  SaturateOnIntegerOverflow=on  OutDataTypeStr=Inherit: Same as first input
  Out1 : Outport  VectorParamsAs1DForOutWhenUnconnected=off
  wires:
  Sum1/1 -> Out1/1
  In1/1 -> Sum1/2
  Constant/1 -> Sum1/1

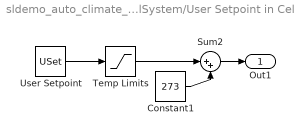
== system sldemo_auto_climate_elec/ClimateControlSystem/User Setpoint in Celsius ==
  Constant1 : Constant  Value=273
  Sum2 : Sum  Inputs=|++  InputSameDT=on  SaturateOnIntegerOverflow=on  OutDataTypeStr=Inherit: Same as first input
  Temp Limits : Saturate  UpperLimit=100  LowerLimit=-99
  User Setpoint : Constant  Value=USet
  Out1 : Outport  VectorParamsAs1DForOutWhenUnconnected=off
  wires:
  Temp Limits/1 -> Sum2/1
  Constant1/1 -> Sum2/2
  User Setpoint/1 -> Temp Limits/1
  Sum2/1 -> Out1/1

== system sldemo_auto_climate_elec/ElectricalSystem/AC Current Sensors ==
  Current Sensor : ee_lib/Sensors & Transducers/Current Sensor (Three-Phase)
  PS-Simulink Converter8 : nesl_utility/PS-Simulink Converter  PhysicalDomain=network_engine_domain  SubClassName=ps_output  LeftPortType=input  RightPortType=output  PseudoPeriodic=off  Frequencies=[]  Unit=1  AffineConversion=off
      settings: SourceProductBaseCode=PW,SS
  Phase Currents : Scope
  ~1 : PMIOPort  Side=Left
  ~2 : PMIOPort  Port=2  Side=Right
  wires:
  PS-Simulink Converter8/1 -> Phase Currents/1
  connections:
  Current Sensor/RConn2 -- ~2/RConn1
  Current Sensor/LConn1 -- ~1/RConn1
  Current Sensor/RConn1 -- PS-Simulink Converter8/LConn1

== system sldemo_auto_climate_elec/ElectricalSystem/DC Current Sensor ==
  " DC Current" : Scope
  Current Sensor4 : fl_lib/Electrical/Electrical Sensors/Current Sensor
  PS-Simulink Converter9 : nesl_utility/PS-Simulink Converter  PhysicalDomain=network_engine_domain  SubClassName=ps_output  LeftPortType=input  RightPortType=output  PseudoPeriodic=off  Frequencies=[]  Unit=1  AffineConversion=off
      settings: SourceProductBaseCode=PW,SS
  - : PMIOPort  Side=Right
  + : PMIOPort  Port=2  Side=Left
  wires:
  PS-Simulink Converter9/1 -> " DC Current"/1
  connections:
  Current Sensor4/LConn1 -- +/RConn1
  Current Sensor4/RConn1 -- PS-Simulink Converter9/LConn1
  Current Sensor4/RConn2 -- -/RConn1

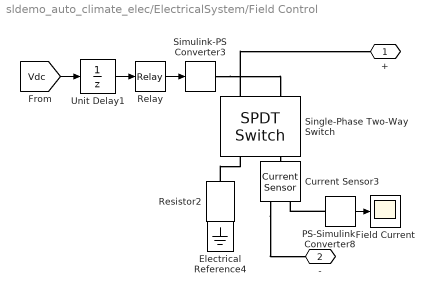
== system sldemo_auto_climate_elec/ElectricalSystem/Field Control ==
  Current Sensor3 : fl_lib/Electrical/Electrical Sensors/Current Sensor
  Electrical Reference4 : fl_lib/Electrical/Electrical Elements/Electrical Reference
  Field Current : Scope
  PS-Simulink Converter8 : nesl_utility/PS-Simulink Converter  PhysicalDomain=network_engine_domain  SubClassName=ps_output  LeftPortType=input  RightPortType=output  PseudoPeriodic=off  Frequencies=[]  Unit=1  AffineConversion=off
      settings: SourceProductBaseCode=PW,SS
  Relay : Relay  OnSwitchValue=14.5  OffSwitchValue=13.5
  Resistor2 : fl_lib/Electrical/Electrical Elements/Resistor  R=1e3 Ohm  i_specify=off  i_priority=None  i=0 A  i_nominal_specify=off  i_nominal_unit=A  i_nominal_value=1  v_specify=off  v_priority=None  v=0 V  v_nominal_specify=off  v_nominal_unit=V  v_nominal_value=1
  Simulink-PS Converter3 : nesl_utility/Simulink-PS Converter  PhysicalDomain=network_engine_domain  SubClassName=ps_input  LeftPortType=input  RightPortType=output  PseudoPeriodic=off  Frequencies=[]  NoiseDistribution=none  NoiseParameters=[]  Unit=1  AffineConversion=off  FilteringAndDerivatives=provide  SimscapeFilterOrder=1  InputFilterTimeConstant=0.001  UdotUserProvided=0
      settings: SourceProductBaseCode=PW,SS
  Single-Phase Two-Way Switch : ee_lib/Switches & Breakers/SPDT Switch  R_closed=0.001 Ohm  G_open=1e-6 1/Ohm  Threshold=0.5 V  Width=0 V  model_dynamics=0  t_on=1e-3 s  t_off=1e-3 s  initial_vT=0 V
      settings: SourceProductBaseCode=PS
  Unit Delay1 : UnitDelay  InitialCondition=12  SampleTime=-1  HasFrameUpgradeWarning=on
  + : PMIOPort  Side=Left
  - : PMIOPort  Port=2  Side=Right
  wires:
  Relay/1 -> Simulink-PS Converter3/1
  PS-Simulink Converter8/1 -> Field Current/1
  [Vdc] -> Unit Delay1/1
  Unit Delay1/1 -> Relay/1
  connections:
  Simulink-PS Converter3/RConn1 -- Single-Phase Two-Way Switch/LConn1
  Electrical Reference4/LConn1 -- Resistor2/RConn1
  Single-Phase Two-Way Switch/RConn1 -- Current Sensor3/LConn1
  Resistor2/LConn1 -- Single-Phase Two-Way Switch/RConn2
  PS-Simulink Converter8/LConn1 -- Current Sensor3/RConn1
  Current Sensor3/RConn2 -- -/RConn1
  Single-Phase Two-Way Switch/LConn2 -- +/RConn1

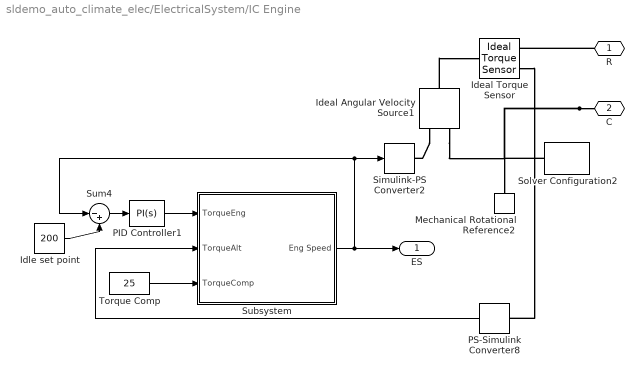
== system sldemo_auto_climate_elec/ElectricalSystem/IC Engine ==
  Ideal Angular Velocity Source1 : fl_lib/Mechanical/Mechanical Sources/Ideal Angular Velocity Source
  Ideal Torque Sensor : fl_lib/Mechanical/Mechanical Sensors/Ideal Torque Sensor
  Idle set point : Constant  Value=200
  Mechanical Rotational Reference2 : fl_lib/Mechanical/Rotational Elements/Mechanical Rotational Reference
  PID Controller1 : slpidlib/PID Controller  Controller=PI  Form=Parallel  TimeDomain=Continuous-time  UseExternalTs=off  SampleTime=-1  IntegratorMethod=Forward Euler  FilterMethod=Forward Euler  ControllerParametersSource=internal  P=2  I=8  D=1  UseFilter=on  N=1000  TunerSelectOption=Transfer Function Based (PID Tuner App)  InitialConditionSource=internal  InitialConditionForIntegrator=0  InitialConditionForFilter=0  DifferentiatorICPrevScaledInput=0  ExternalReset=none  TrackingMode=off  Kt=1  LimitOutput=off  SatLimitsSource=internal  UpperSaturationLimit=inf  LowerSaturationLimit=-inf  LinearizeAsGain=on  AntiWindupMode=none  Kb=1  POutMin=[]  POutMax=[]  IOutMin=[]  IOutMax=[]  DOutMin=[]  DOutMax=[]  NOutMin=[]  NOutMax=[]  SumOutMin=[]  SumOutMax=[]  SaturationOutMin=[]  SaturationOutMax=[]  PParamMin=[]  PParamMax=[]  IParamMin=[]  IParamMax=[]  DParamMin=[]  DParamMax=[]  NParamMin=[]  NParamMax=[]  KbParamMin=[]  KbParamMax=[]  KtParamMin=[]  KtParamMax=[]  KbOutMin=[]  KbOutMax=[]  KtOutMin=[]  KtOutMax=[]  IntegratorOutMin=[]  IntegratorOutMax=[]  FilterOutMin=[]  FilterOutMax=[]  SumI1OutMin=[]  SumI1OutMax=[]  SumI2OutMin=[]  SumI2OutMax=[]  SumI3OutMin=[]  SumI3OutMax=[]  SumI4OutMin=[]  SumI4OutMax=[]  SumDOutMin=[]  SumDOutMax=[]  DifferentiatorOutMin=[]  DifferentiatorOutMax=[]  FilterDiffOutCoefMin=[]  FilterDiffOutCoefMax=[]  ReciprocalOutMin=[]  ReciprocalOutMax=[]  SumDenOutMin=[]  SumDenOutMax=[]  SumNumOutMin=[]  SumNumOutMax=[]  DivideOutMin=[]  DivideOutMax=[]  UdiffTsProdOutMin=[]  UdiffTsProdOutMax=[]  NTsProdOutMin=[]  NTsProdOutMax=[]  UintegralTsProdOutMin=[]  UintegralTsProdOutMax=[]  UngainTsProdOutMin=[]  UngainTsProdOutMax=[]  IntegratorContinuousStateAttributes=''  IntegratorStateMustResolveToSignalObject=off  IntegratorRTWStateStorageClass=Auto  FilterContinuousStateAttributes=''  FilterStateMustResolveToSignalObject=off  FilterRTWStateStorageClass=Auto  ParallelPVariant=InternalParameters  IdealPVariant=Disabled  IVariant=InternalParameters  DVariant=Disabled  IntegratorVariant=Continuous  SatVariant=Disabled  AWVariant=Passthrough  PCopyVariant=Disabled  TRVariant=Disabled  FdbkBlocksVariant=Forward  IdealPFdbkVariant=Disabled  SatFdbkVariant=Disabled  DerivativeFilterVariant=Disabled  NVariant=Disabled  NCopyVariant=Disabled_SignalSpec  FilterICVariant=Disabled  IntegratorICVariant=InternalICs  ExternalResetVariant=Disabled  TRSumVariant=Passthrough  SumFdbkVariant=Disabled  SumVariant=Sum_PI  TsampFilterVariant=InternalTs  TsampNgainVariant=Passthrough  TsampIntegralVariant=Passthrough  ExternalSaturationOutDataTypeStr=Inherit: Same as second input
  PS-Simulink Converter8 : nesl_utility/PS-Simulink Converter  PhysicalDomain=network_engine_domain  SubClassName=ps_output  LeftPortType=input  RightPortType=output  PseudoPeriodic=off  Frequencies=[]  Unit=1  AffineConversion=off
      settings: SourceProductBaseCode=PW,SS
  Simulink-PS Converter2 : nesl_utility/Simulink-PS Converter  PhysicalDomain=network_engine_domain  SubClassName=ps_input  LeftPortType=input  RightPortType=output  PseudoPeriodic=off  Frequencies=[]  NoiseDistribution=none  NoiseParameters=[]  Unit=1  AffineConversion=off  FilteringAndDerivatives=provide  SimscapeFilterOrder=1  InputFilterTimeConstant=0.001  UdotUserProvided=0
      settings: SourceProductBaseCode=PW,SS
  Solver Configuration2 : nesl_utility/Solver Configuration  PhysicalDomain=network_engine_domain  SubClassName=solver  LeftPortType=input  RightPortType=generic  Tones=[]  Harmonics=[]  SimulateNoise=off  Profile=off  UseLocalSampling=off  EnableSwitchedLinearOptims=on  FrequencyDomain=off  UseCCode=off  RelTol=0.001  AbsTol=1e-06  MinStep=1e-09  ToWorkspace=off  RevertToSquareIcSolve=off  NumHomotopyIterations=100  PhasorMode=off  PhasorModeNumHarmonics=1  DoDC=off  ResidualTolerance=1e-09  UseLocalSolver=on  LocalSolverChoice=NE_BACKWARD_EULER_ADVANCER  LocalSolverSampleTime=1e-5  DoFixedCost=on  MaxNonlinIter=4  MaxModeIter=2  ComputeImpulses=off  ImpulseIterations=2  LinearAlgebra=Sparse  EquationFormulation=NE_TIME_EF  DelaysMemoryBudget=1024  AutomaticFiltering=on  FilteringTimeConstant=0.001  PartitionStorageMethod=AS_NEEDED  PartitionMemoryBudget=1024  PartitionMethod=FAST
      settings: SourceProductBaseCode=PW,SS
  Subsystem : Subsystem
  Sum4 : Sum  Inputs=|-+  InputSameDT=on  SaturateOnIntegerOverflow=on  OutDataTypeStr=Inherit: Same as first input
  Torque Comp : Constant  Value=25
  R : PMIOPort  Side=Left
  C : PMIOPort  Port=2  Side=Right
  ES : Outport  InitialOutput=0  VectorParamsAs1DForOutWhenUnconnected=off
  wires:
  Subsystem/1(Eng Speed) -> Sum4/1, Simulink-PS Converter2/1, ES/1
  Torque Comp/1 -> Subsystem/3(TorqueComp)
  PS-Simulink Converter8/1 -> Subsystem/2(TorqueAlt)
  Sum4/1 -> PID Controller1/1
  Idle set point/1 -> Sum4/2
  PID Controller1/1 -> Subsystem/1(TorqueEng)
  connections:
  Ideal Angular Velocity Source1/LConn1 -- Ideal Torque Sensor/LConn1
  Ideal Torque Sensor/RConn2 -- PS-Simulink Converter8/LConn1
  Ideal Angular Velocity Source1/RConn1 -- Simulink-PS Converter2/RConn1
  R/RConn1 -- Ideal Torque Sensor/RConn1
  C/RConn1 -- Ideal Angular Velocity Source1/RConn2 -- Mechanical Rotational Reference2/LConn1 -- Solver Configuration2/RConn1

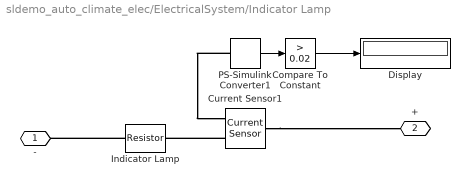
== system sldemo_auto_climate_elec/ElectricalSystem/Indicator Lamp ==
  Compare To Constant : simulink/Logic and Bit Operations/Compare To Constant  relop=>  const=0.02  OutDataTypeStr=boolean
  Current Sensor1 : fl_lib/Electrical/Electrical Sensors/Current Sensor
  Display : Display
  Indicator Lamp : fl_lib/Electrical/Electrical Elements/Resistor  R=10 Ohm  i_specify=off  i_priority=None  i=0 A  i_nominal_specify=off  i_nominal_unit=A  i_nominal_value=1  v_specify=off  v_priority=None  v=0 V  v_nominal_specify=off  v_nominal_unit=V  v_nominal_value=1
  PS-Simulink Converter1 : nesl_utility/PS-Simulink Converter  PhysicalDomain=network_engine_domain  SubClassName=ps_output  LeftPortType=input  RightPortType=output  PseudoPeriodic=off  Frequencies=[]  Unit=1  AffineConversion=off
      settings: SourceProductBaseCode=PW,SS
  - : PMIOPort  Side=Left
  + : PMIOPort  Port=2  Side=Right
  wires:
  Compare To Constant/1 -> Display/1
  PS-Simulink Converter1/1 -> Compare To Constant/1
  connections:
  Current Sensor1/RConn2 -- Indicator Lamp/RConn1
  Indicator Lamp/LConn1 -- -/RConn1
  PS-Simulink Converter1/LConn1 -- Current Sensor1/RConn1
  Current Sensor1/LConn1 -- +/RConn1

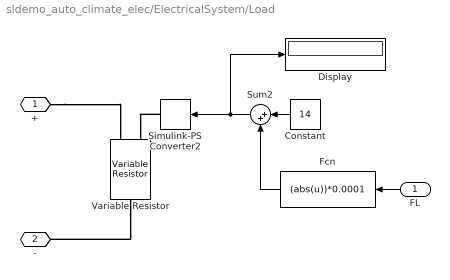
== system sldemo_auto_climate_elec/ElectricalSystem/Load ==
  FL : Inport
  Constant : Constant  Value=14
  Display : Display
  Fcn : Fcn  Expr=(abs(u))*0.0001
  Simulink-PS Converter2 : nesl_utility/Simulink-PS Converter  PhysicalDomain=network_engine_domain  SubClassName=ps_input  LeftPortType=input  RightPortType=output  PseudoPeriodic=off  Frequencies=[]  NoiseDistribution=none  NoiseParameters=[]  Unit=1  AffineConversion=off  FilteringAndDerivatives=provide  SimscapeFilterOrder=1  InputFilterTimeConstant=0.001  UdotUserProvided=0
      settings: SourceProductBaseCode=PW,SS
  Sum2 : Sum  Inputs=|++  InputSameDT=on  SaturateOnIntegerOverflow=on  OutDataTypeStr=Inherit: Same as first input
  Variable Resistor : fl_lib/Electrical/Electrical Elements/Variable Resistor  Rmin=0.1 Ohm  i_specify=off  i_priority=None  i=0 A  i_nominal_specify=off  i_nominal_unit=A  i_nominal_value=1  v_specify=off  v_priority=None  v=0 V  v_nominal_specify=off  v_nominal_unit=V  v_nominal_value=1
  + : PMIOPort  Side=Left
  - : PMIOPort  Port=2  Side=Right
  wires:
  Sum2/1 -> Simulink-PS Converter2/1, Display/1
  Fcn/1 -> Sum2/2
  Constant/1 -> Sum2/1
  FL/1 -> Fcn/1
  connections:
  Simulink-PS Converter2/RConn1 -- Variable Resistor/LConn1
  Variable Resistor/RConn1 -- -/RConn1
  +/RConn1 -- Variable Resistor/LConn2

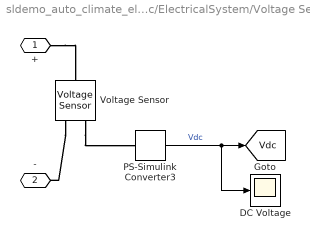
== system sldemo_auto_climate_elec/ElectricalSystem/Voltage Sensor ==
  DC Voltage : Scope
  PS-Simulink Converter3 : nesl_utility/PS-Simulink Converter  PhysicalDomain=network_engine_domain  SubClassName=ps_output  LeftPortType=input  RightPortType=output  PseudoPeriodic=off  Frequencies=[]  Unit=1  AffineConversion=off
      settings: SourceProductBaseCode=PW,SS
  Voltage Sensor : fl_lib/Electrical/Electrical Sensors/Voltage Sensor
  + : PMIOPort  Side=Left
  - : PMIOPort  Port=2  Side=Right
  tag scope: Vdc=global
  wires:
  PS-Simulink Converter3/1 -> DC Voltage/1, [Vdc]  "Vdc"
  connections:
  Voltage Sensor/RConn1 -- PS-Simulink Converter3/LConn1
  Voltage Sensor/RConn2 -- -/RConn1
  +/RConn1 -- Voltage Sensor/LConn1

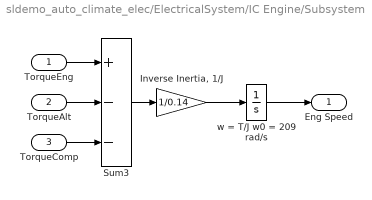
== system sldemo_auto_climate_elec/ElectricalSystem/IC Engine/Subsystem ==
  TorqueEng : Inport
  TorqueAlt : Inport  Port=2
  TorqueComp : Inport  Port=3
  "Inverse Inertia, 1/J" : Gain  Gain=1/0.14  SaturateOnIntegerOverflow=on  OutDataTypeStr=Inherit: Same as input  ParamDataTypeStr=Inherit: Same as input
  Sum3 : Sum  Inputs=+--  InputSameDT=on  SaturateOnIntegerOverflow=on  OutDataTypeStr=Inherit: Same as first input
  w = T/J w0 = 209 rad/s : Integrator  InitialCondition=209.48  ZeroCross=off
  Eng Speed : Outport  InitialOutput=0  VectorParamsAs1DForOutWhenUnconnected=off
  wires:
  w = T/J w0 = 209 rad/s/1 -> Eng Speed/1
  TorqueComp/1 -> Sum3/3
  TorqueAlt/1 -> Sum3/2
  TorqueEng/1 -> Sum3/1
  Sum3/1 -> "Inverse Inertia, 1/J"/1
  "Inverse Inertia, 1/J"/1 -> w = T/J w0 = 209 rad/s/1
